simulink model "linear_model"  (R2021b)
settings: Solver=VariableStepAuto  StartTime=0.0  StopTime=10.0  RelTol=1e-3
undefined symbols (not defined in the file or in its folder): A, B, C, D
libraries: simulink x1
settings Model: Creator=lara  LastModifiedBy=lara

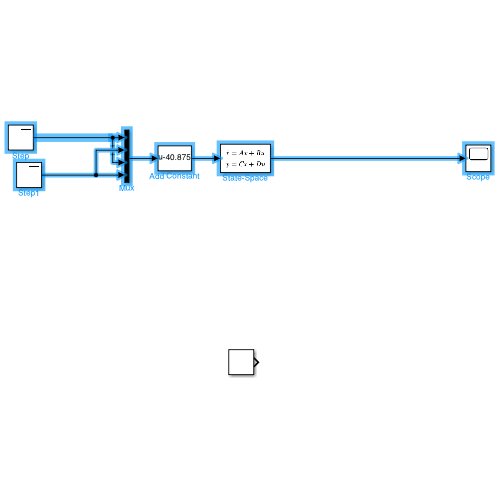
[thumbnail: Simulink's stored preview of the top-level diagram]
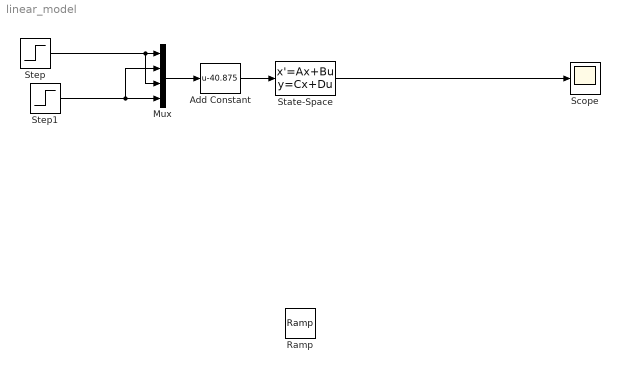
== system linear_model ==
  Add Constant : Bias  Bias=-40.875
  Mux : Mux
  Ramp : simulink/Sources/Ramp  slope=1  start=0  InitialOutput=0
  Scope : Scope
  State-Space : StateSpace  A=A  B=B  C=C  D=D  InitialCondition=zeros(1,12)
  Step : Step  Time=0  After=5+40.875  SampleTime=0
  Step1 : Step  Time=0  After=5+40.875  SampleTime=0
  wires:
  State-Space/1 -> Scope/1
  Mux/1 -> Add Constant/1
  Add Constant/1 -> State-Space/1
  Step/1 -> Mux/3, Mux/1
  Step1/1 -> Mux/2, Mux/4
